simulink model "EvitaParedes"  (R2023b)
settings: Solver=FixedStepAuto  StartTime=0.0  StopTime=inf  RelTol=1e-3  EnableMultiTasking=on
libraries: simulink x3
settings Model: ExtModeTrigDuration=2  Creator=chaya  LastModifiedBy=chaya
settings OptimizationCC: EnhancedBackFolding=on  PassReuseOutputArgsAs=Individual arguments  ZeroExternalMemoryAtStartup=off  ZeroInternalMemoryAtStartup=off  MaxStackSize=64  OptimizeBlockOrder=speed  DifferentSizesBufferReuse=on  OptimizationCustomize=off  EfficientTunableParamExpr=on
settings DebuggingCC: ParameterOverflowMsg=none  ParameterTunabilityLossMsg=error
settings HardwareCC: ProdBitPerInt=16  ProdBitPerPointer=16  ProdBitPerSizeT=16  ProdBitPerPtrDiffT=16  ProdLargestAtomicFloat=None  ProdWordSize=8  ProdHWDeviceType=Atmel->AVR  UseEmbeddedCoderFeatures=off  UseSimulinkCoderFeatures=off
settings SFSimCC: MATLABDynamicMemAlloc=off
settings RTWCC: Description=Embedded Coder  SystemTargetFile=ert.tlc  HardwareBoard=Arduino Mega 2560  TemplateMakefile=ert_default_tmf  Toolchain=Arduino AVR  BuildConfiguration=Faster Runs
settings CodeAppCC: ForceParamTrailComments=on  IgnoreCustomStorageClasses=off  OperatorAnnotations=on  SimulinkDataObjDesc=on  SFDataObjDesc=on  InsertBlockDesc=on
settings ERTTargetCC: SupportContinuousTime=on  SupportNonInlinedSFcns=on  SupportVariableSizeSignals=on  ExtModeTransport=3  ExtModeStaticAlloc=on  ExtModeAutomaticAllocSize=off  ExtModeStaticAllocSize=2048  ExtModeMexFile=ext_xcp  ExtModeIntrfLevel=Level2 - Open

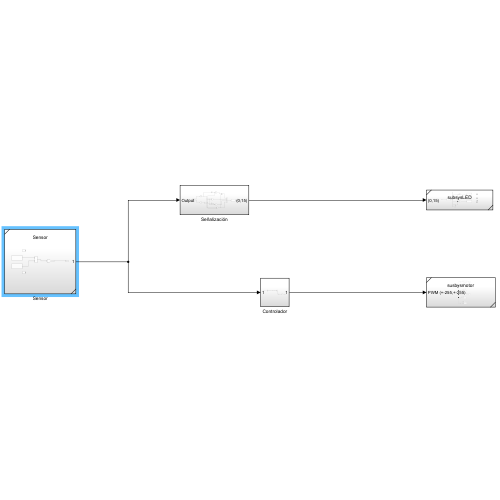
[thumbnail: Simulink's stored preview of the top-level diagram]
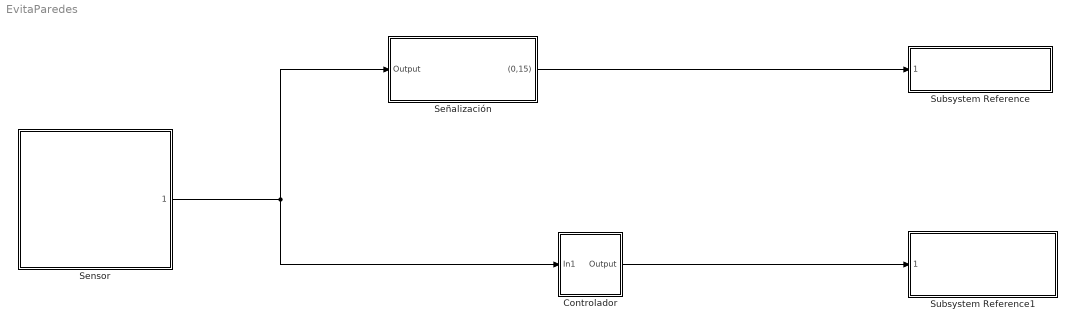
== system EvitaParedes ==
  Controlador : Subsystem
  Sensor : Subsystem  ReferencedSubsystem=Sensor
  Señalización : Subsystem
  Subsystem Reference : Subsystem  ReferencedSubsystem=subsysLED
  Subsystem Reference1 : Subsystem  ReferencedSubsystem=susbysmotor
  wires:
  Controlador/1(Output) -> Subsystem Reference1/1
  Señalización/1((0,15)) -> Subsystem Reference/1
  Sensor/1 -> Controlador/1(In1), Señalización/1(Output)

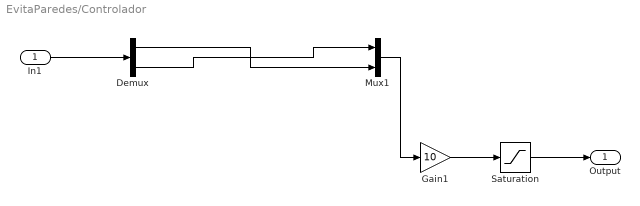
== system EvitaParedes/Controlador ==
  In1 : Inport
  Demux : Demux  Outputs=2
  Gain1 : Gain  Gain=10
  Mux1 : Mux  Inputs=2
  Saturation : Saturate  UpperLimit=255  LowerLimit=-255
  Output : Outport
  wires:
  Gain1/1 -> Saturation/1
  Mux1/1 -> Gain1/1
  Demux/2 -> Mux1/1
  Demux/1 -> Mux1/2
  In1/1 -> Demux/1
  Saturation/1 -> Output/1

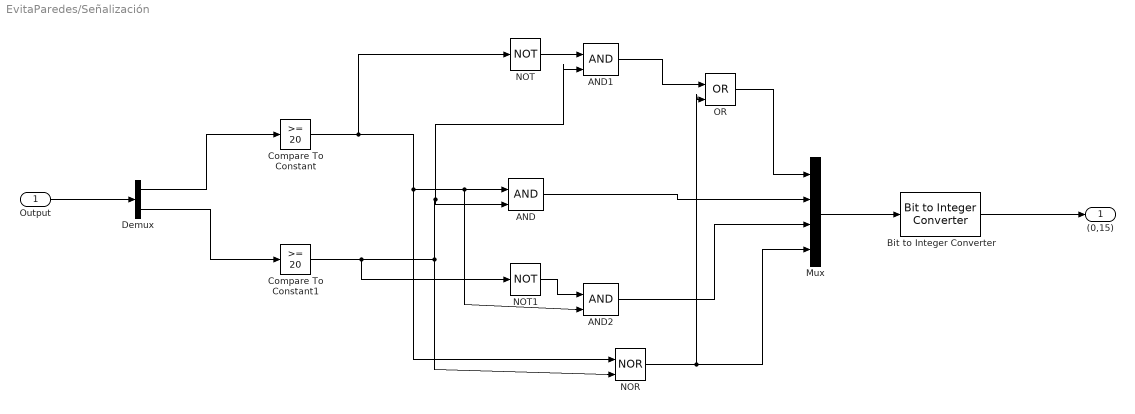
== system EvitaParedes/Señalización ==
  Output : Inport
  AND : Logic  IconShape=distinctive  AllPortsSameDT=off  OutDataTypeStr=boolean
  AND1 : Logic  IconShape=distinctive  AllPortsSameDT=off  OutDataTypeStr=boolean
  AND2 : Logic  IconShape=distinctive  AllPortsSameDT=off  OutDataTypeStr=boolean
  Bit to Integer Converter : simulink/Logic and Bit Operations/Bit to Integer Converter  nbits=4  bitOrder=MSB first  signedOutputValues=Unsigned  outDtype=Inherit via internal rule  outDtypeSigned=Inherit via internal rule
  Compare To Constant : simulink/Logic and Bit Operations/Compare To Constant  relop=>=  const=20  OutDataTypeStr=boolean
  Compare To Constant1 : simulink/Logic and Bit Operations/Compare To Constant  relop=>=  const=20  OutDataTypeStr=boolean
  Demux : Demux  Outputs=2
  Mux : Mux
  NOR : Logic  Operator=NOR  IconShape=distinctive  AllPortsSameDT=off  OutDataTypeStr=boolean
  NOT : Logic  Operator=NOT  IconShape=distinctive  AllPortsSameDT=off  OutDataTypeStr=boolean
  NOT1 : Logic  Operator=NOT  IconShape=distinctive  AllPortsSameDT=off  OutDataTypeStr=boolean
  OR : Logic  Operator=OR  IconShape=distinctive  AllPortsSameDT=off  OutDataTypeStr=boolean
  (0,15) : Outport
  wires:
  Output/1 -> Demux/1
  Demux/1 -> Compare To Constant/1
  Demux/2 -> Compare To Constant1/1
  Compare To Constant/1 -> NOT/1, NOR/1, AND/1, AND2/2
  Compare To Constant1/1 -> NOT1/1, NOR/2, AND1/2, AND/2
  AND/1 -> Mux/2
  NOT/1 -> AND1/1
  NOT1/1 -> AND2/1
  AND2/1 -> Mux/3
  NOR/1 -> OR/2, Mux/4
  AND1/1 -> OR/1
  OR/1 -> Mux/1
  Mux/1 -> Bit to Integer Converter/1
  Bit to Integer Converter/1 -> (0,15)/1
